simulink model "MVB4threeTest"  (R2015a)
settings: Solver=FixedStepDiscrete  SolverMode=SingleTasking  StartTime=0  StopTime=8000  RelTol=1e-3
model workspace (MAT data in the model file):
  logicAddr = 2
settings Model: Creator=qiji  LastModifiedBy=qiji
settings DataIOCC: SignalLoggingSaveFormat=ModelDataLogs
settings OptimizationCC: BlockReduction=off  ConditionallyExecuteInputs=off  InlineParams=on
settings DebuggingCC: SolverPrmCheckMsg=warning  MultiTaskDSMMsg=warning  MultiTaskCondExecSysMsg=none  SingleTaskRateTransMsg=error  SFUnusedDataAndEventsDiag=none

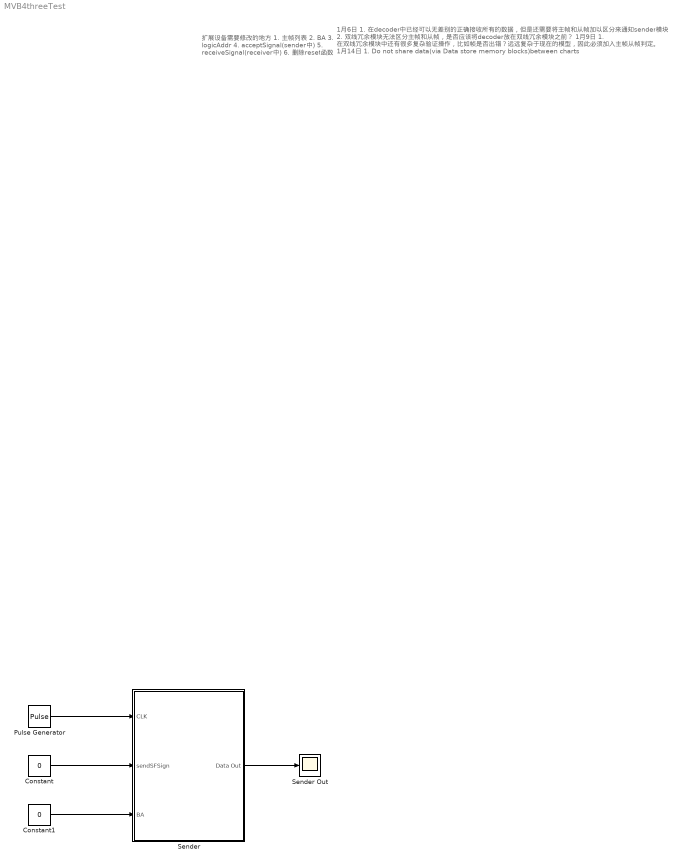
== system MVB4threeTest ==
  note: 扩展设备需要修改的地方
      | 1. 主帧列表
      | 2. BA
      | 3. logicAddr
      | 4. acceptSignal(sender中)
      | 5. receiveSignal(receiver中)
      | 6. 删除reset函数
  note: 1月6日
      | 1. 在decoder中已经可以无差别的正确接收所有的数据，但是还需要将主帧和从帧加以区分来通知sender模块
      | 2. 双线冗余模块无法区分主帧和从帧，是否应该将decoder放在双线冗余模块之前？
      | 1月9日
      | 1. 在双线冗余模块中还有很多复杂验证操作，比如帧是否出错？远远复杂于现在的模型，因此必须加入主帧从帧判定。
      | 1月14日
      | 1. Do not share data(via Data store memory blocks)between charts
  Constant : Constant  Value=0
  Constant1 : Constant  Value=0
  Pulse Generator : DiscretePulseGenerator  Amplitude=true
  Sender : Subsystem
  Sender Out : Scope
  wires:
  Pulse Generator/1 -> Sender/1(CLK)
  Sender/1(Data Out) -> Sender Out/1
  Constant/1 -> Sender/2(sendSFSign)
  Constant1/1 -> Sender/3(BA)

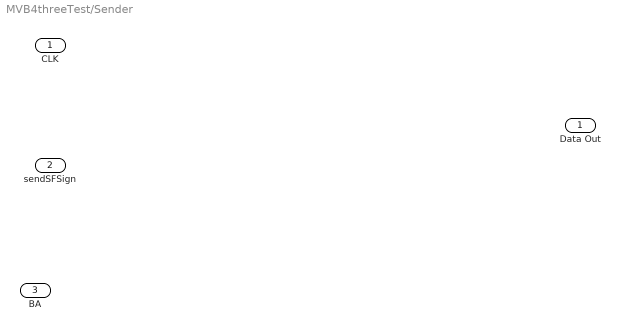
== system MVB4threeTest/Sender ==
  CLK : Inport
  sendSFSign : Inport  Port=2
  BA : Inport  Port=3
  Data Out : Outport
